simulink model "dq_req"  (R2017b)
settings: Solver=VariableStepAuto  StartTime=0.0  StopTime=10.0  RelTol=1e-3
libraries: dspmtrx3 x1
settings Model: Creator=shriyahazra  LastModifiedBy=shriyahazra

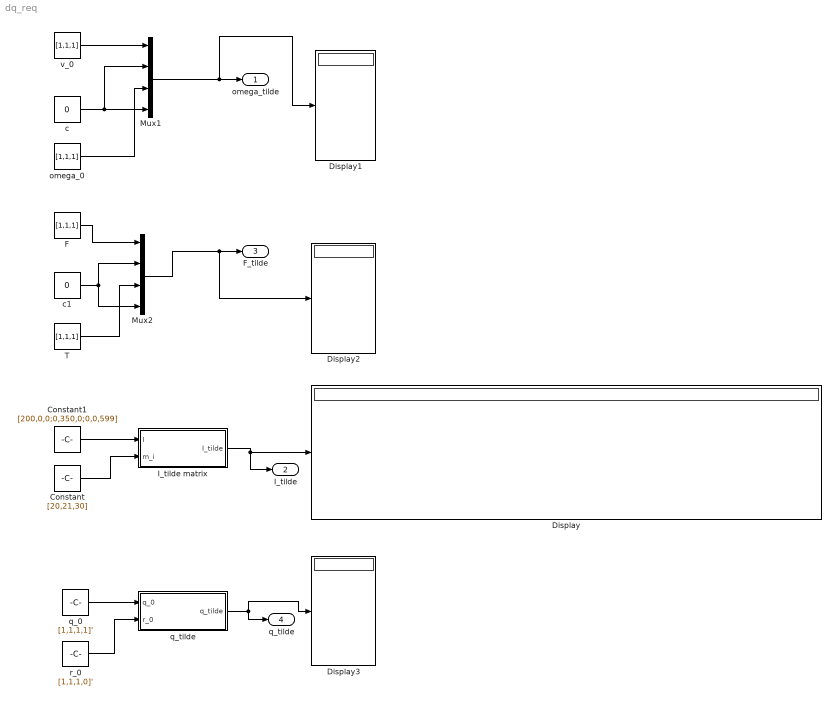
== system dq_req ==
  Constant : Constant  Value=[20,21,30]
  Constant1 : Constant  Value=[200,0,0;0,350,0;0,0,599]
  Display{,1..3} (4 alike) : Display
  F : Constant  Value=[1,1,1]  VectorParams1D=off
  I_tilde matrix : Subsystem
  Mux1 : Mux
  Mux2 : Mux
  T : Constant  Value=[1,1,1]  VectorParams1D=off
  c : Constant  Value=0
  c1 : Constant  Value=0
  omega_0 : Constant  Value=[1,1,1]  VectorParams1D=off
  q_0 : Constant  Value=[1,1,1,1]'  VectorParams1D=off
  "q_tilde " : Subsystem
  r_0 : Constant  Value=[1,1,1,0]'  VectorParams1D=off
  v_0 : Constant  Value=[1,1,1]  VectorParams1D=off
  omega_tilde : Outport
  I_tilde : Outport  Port=2
  F_tilde : Outport  Port=3
  q_tilde : Outport  Port=4
  wires:
  Constant/1 -> I_tilde matrix/2(m_i)
  Constant1/1 -> I_tilde matrix/1(I)
  I_tilde matrix/1(I_tilde) -> I_tilde/1, Display/1
  Mux1/1 -> Display1/1, omega_tilde/1
  omega_0/1 -> Mux1/3
  v_0/1 -> Mux1/1
  c/1 -> Mux1/4, Mux1/2
  F/1 -> Mux2/1
  c1/1 -> Mux2/4, Mux2/2
  T/1 -> Mux2/3
  Mux2/1 -> F_tilde/1, Display2/1
  q_0/1 -> "q_tilde "/1(q_0)
  r_0/1 -> "q_tilde "/2(r_0)
  "q_tilde "/1(q_tilde) -> q_tilde/1, Display3/1

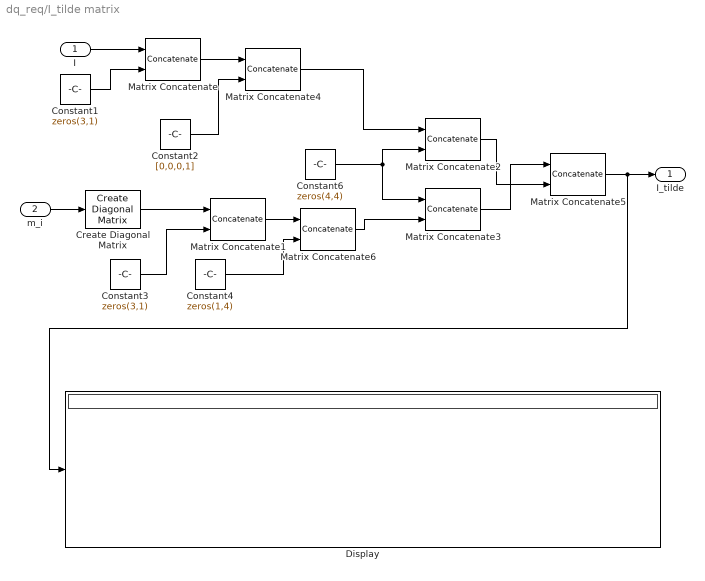
== system dq_req/I_tilde matrix ==
  I : Inport
  m_i : Inport  Port=2
  Constant1 : Constant  Value=zeros(3,1)  VectorParams1D=off
  Constant2 : Constant  Value=[0,0,0,1]  VectorParams1D=off
  Constant3 : Constant  Value=zeros(3,1)  VectorParams1D=off
  Constant4 : Constant  Value=zeros(1,4)  VectorParams1D=off
  Constant6 : Constant  Value=zeros(4,4)
  Create Diagonal Matrix : dspmtrx3/Create Diagonal Matrix
      settings: SourceProductName=DSP System Toolbox  SourceProductBaseCode=DS
  Display : Display
  Matrix Concatenate{,1..3} (4 alike) : Concatenate  Mode=Multidimensional array  ConcatenateDimension=2
  Matrix Concatenate4 : Concatenate  Mode=Multidimensional array
  Matrix Concatenate5 : Concatenate  Mode=Multidimensional array
  Matrix Concatenate6 : Concatenate  Mode=Multidimensional array
  I_tilde : Outport
  wires:
  Matrix Concatenate5/1 -> Display/1, I_tilde/1
  Matrix Concatenate2/1 -> Matrix Concatenate5/2
  Matrix Concatenate3/1 -> Matrix Concatenate5/1
  Constant1/1 -> Matrix Concatenate/2
  I/1 -> Matrix Concatenate/1
  Constant2/1 -> Matrix Concatenate4/2
  Matrix Concatenate4/1 -> Matrix Concatenate2/1
  Matrix Concatenate/1 -> Matrix Concatenate4/1
  m_i/1 -> Create Diagonal Matrix/1
  Constant3/1 -> Matrix Concatenate1/2
  Matrix Concatenate6/1 -> Matrix Concatenate3/2
  Create Diagonal Matrix/1 -> Matrix Concatenate1/1
  Constant6/1 -> Matrix Concatenate3/1, Matrix Concatenate2/2
  Constant4/1 -> Matrix Concatenate6/2
  Matrix Concatenate1/1 -> Matrix Concatenate6/1

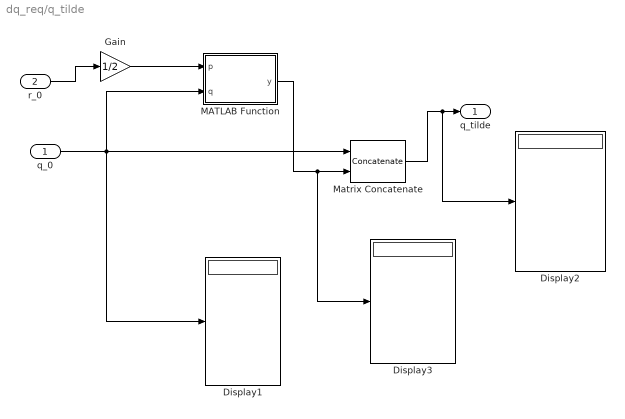
== system dq_req/q_tilde  ==
  q_0 : Inport
  r_0 : Inport  Port=2
  Display1 : Display
  Display2 : Display
  Display3 : Display
  Gain : Gain  Gain=1/2
  MATLAB Function : MATLAB Function  TreatAsAtomicUnit=on
  Matrix Concatenate : Concatenate  Mode=Multidimensional array
  q_tilde : Outport
  wires:
  Matrix Concatenate/1 -> Display2/1, q_tilde/1
  r_0/1 -> Gain/1
  Gain/1 -> MATLAB Function/1(p)
  q_0/1 -> Display1/1, MATLAB Function/2(q), Matrix Concatenate/1
  MATLAB Function/1(y) -> Display3/1, Matrix Concatenate/2

== matlab function dq_req/q_tilde /MATLAB Function ==
  data: p input; y output; q input
function y = quat_mult(p,q)

pvect= p(1:3);
p4= p(4);

qvect= q(1:3);
q4= q(4);

y = [q4.*pvect + p4.*qvect - cross(pvect, qvect); p4*q4 - sum(pvect.*qvect,1)];
